simulink model "orientation_box"  (R2019b)
settings: Solver=ode45  StartTime=0.0  StopTime=20000.0  MaxStep=0.01  RelTol=1e-8
settings Model: Creator=Hector  LastModifiedBy=Hector

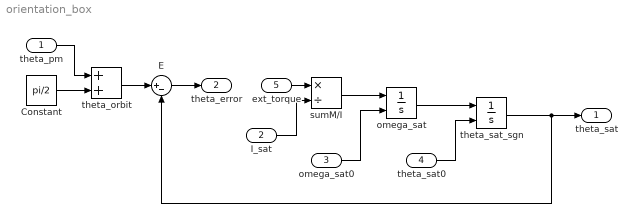
== system orientation_box ==
  theta_pm : Inport
  I_sat : Inport  Port=2
  omega_sat0 : Inport  Port=3
  theta_sat0 : Inport  Port=4
  ext_torque : Inport  Port=5
  Constant : Constant  Value=pi/2
  E : Sum  Inputs=|+-
  omega_sat : Integrator  InitialConditionSource=external  InitialCondition=pi/30
  sumM/I : Product  Inputs=*/
  theta_orbit : Sum
  theta_sat_sgn : Integrator  InitialConditionSource=external  InitialCondition=pi/6
  theta_sat : Outport
  theta_error : Outport  Port=2
  wires:
  ext_torque/1 -> sumM/I/1
  I_sat/1 -> sumM/I/2
  sumM/I/1 -> omega_sat/1
  omega_sat/1 -> theta_sat_sgn/1
  theta_sat_sgn/1 -> theta_sat/1, E/2
  E/1 -> theta_error/1
  theta_orbit/1 -> E/1
  Constant/1 -> theta_orbit/2
  theta_pm/1 -> theta_orbit/1
  omega_sat0/1 -> omega_sat/2
  theta_sat0/1 -> theta_sat_sgn/2
